simulink model "Opgavemodel"  (R2024a)
settings: Solver=VariableStepAuto  StartTime=0.0  StopTime=10.0  RelTol=1e-3
values from neighbouring files (symbols this model uses):
  A = [0 1; 0 -alpha]    [Kladefil.m]    (also in Opgaver.m = [-15 -6.75 -2.5)
  Ac = [A-K.*B-C.*L         Ke*B ... (first row only)    [Opgaver.m]
  B = [0;1]    [Kladefil.m]    (also in Opgaver.m = [8)
  Bc = [Bc transpose(L)]    [Opgaver.m]
  C = [K2 0]    [Kladefil.m]    (also in Opgaver.m = [0 1.5625 3.9063])
  Cc = [-K Ke]    [Opgaver.m]
settings Model: Creator=jesperbertelsen  LastModifiedBy=jesperbertelsen

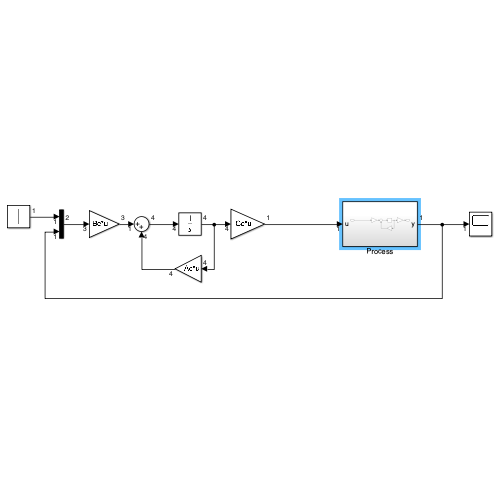
[thumbnail: Simulink's stored preview of the top-level diagram]
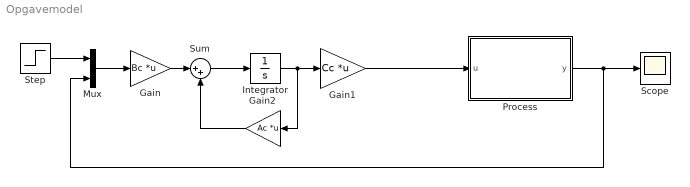
== system Opgavemodel ==
  Gain : Gain  Gain=Bc  Multiplication=Matrix(K*u)
  Gain1 : Gain  Gain=Cc  Multiplication=Matrix(K*u)
  Gain2 : Gain  Gain=Ac  Multiplication=Matrix(K*u)
  Integrator : Integrator
  Mux : Mux  Inputs=2
  Process : Subsystem
  Scope : Scope
  Step : Step  SampleTime=0
  Sum : Sum  Inputs=|++
  wires:
  Gain/1 -> Sum/1
  Sum/1 -> Integrator/1
  Integrator/1 -> Gain2/1, Gain1/1
  Gain2/1 -> Sum/2
  Step/1 -> Mux/1
  Mux/1 -> Gain/1
  Gain1/1 -> Process/1(u)
  Process/1(y) -> Mux/2, Scope/1

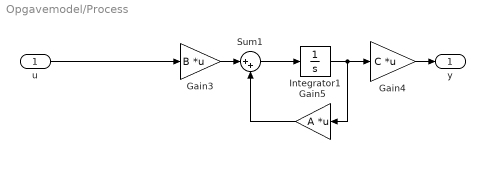
== system Opgavemodel/Process ==
  u : Inport
  Gain3 : Gain  Gain=B  Multiplication=Matrix(K*u)
  Gain4 : Gain  Gain=C  Multiplication=Matrix(K*u)
  Gain5 : Gain  Gain=A  Multiplication=Matrix(K*u)
  Integrator1 : Integrator
  Sum1 : Sum  Inputs=|++
  y : Outport
  wires:
  Gain4/1 -> y/1
  u/1 -> Gain3/1
  Sum1/1 -> Integrator1/1
  Gain3/1 -> Sum1/1
  Integrator1/1 -> Gain5/1, Gain4/1
  Gain5/1 -> Sum1/2
